simulink model "ClosedLoop_Kernel_RBMCntrl_1A"  (R2023b)
settings: Solver=ode4  StartTime=0.0  StopTime=TMax  FixedStep=DT  MaxStep=DT  RelTol=1e-3  EnableMultiTasking=on
values from neighbouring files (symbols this model uses):
  AirfoilCommand = zeros(1,3)'    [openFASTinit.m]    (also in openFASTinit_v2.m)
  Azimuth_index = 1    [openFASTinit.m]    (also in openFASTinit_v2.m)
  B1N1Alpha_index = 1    [openFASTinit.m]    (also in openFASTinit_v2.m)
  B1N1Cl_index = 1    [openFASTinit.m]    (also in openFASTinit_v2.m)
  B1N1Fl_index = 1    [openFASTinit.m]    (also in openFASTinit_v2.m)
  B1N2Fl_index = 1    [openFASTinit.m]    (also in openFASTinit_v2.m)
  B1N3Fl_index = 1    [openFASTinit.m]    (also in openFASTinit_v2.m)
  B2N1Cl_index = 1    [openFASTinit.m]    (also in openFASTinit_v2.m)
  B2N1Fl_index = 1    [openFASTinit.m]    (also in openFASTinit_v2.m)
  B2N2Fl_index = 1    [openFASTinit.m]    (also in openFASTinit_v2.m)
  B2N3Fl_index = 1    [openFASTinit.m]    (also in openFASTinit_v2.m)
  B3N1Cl_index = 1    [openFASTinit.m]    (also in openFASTinit_v2.m)
  B3N1Fl_index = 1    [openFASTinit.m]    (also in openFASTinit_v2.m)
  B3N2Fl_index = 1    [openFASTinit.m]    (also in openFASTinit_v2.m)
  B3N3Fl_index = 1    [openFASTinit.m]    (also in openFASTinit_v2.m)
  BldPitch1_index = 1    [openFASTinit.m]    (also in openFASTinit_v2.m)
  BldPitch2_index = 1    [openFASTinit.m]    (also in openFASTinit_v2.m)
  BldPitch3_index = 1    [openFASTinit.m]    (also in openFASTinit_v2.m)
  CableDelta_Commande = zeros(1,20)'    [openFASTinit.m]    (also in openFASTinit_v2.m)
  CableDelta_dot_Commande = zeros(1,20)'    [openFASTinit.m]    (also in openFASTinit_v2.m)
  DT = str2double((cell_.Cell_line_1))    [Parameters_checking.m]
  ElectTorque = 1000    [openFASTinit.m]    (also in openFASTinit_v2.m = 500)
  GenPwr_index = 1    [openFASTinit.m]    (also in openFASTinit_v2.m)
  GenTorque = 1000    [openFASTinit.m]    (also in openFASTinit_v2.m = 800)
  GenTq_index = 1    [openFASTinit.m]    (also in openFASTinit_v2.m)
  h_sam = block.InputPort(7).Data    [PMC_kernel.m]
  PtfmPitch_index = 1    [openFASTinit.m]    (also in openFASTinit_v2.m)
  PtfmRoll_index = 1    [openFASTinit.m]    (also in openFASTinit_v2.m)
  PtfmYaw_index = 1    [openFASTinit.m]    (also in openFASTinit_v2.m)
  RootMyb1_index = 1    [openFASTinit.m]    (also in openFASTinit_v2.m)
  RootMyb2_index = 1    [openFASTinit.m]    (also in openFASTinit_v2.m)
  RootMyb3_index = 1    [openFASTinit.m]    (also in openFASTinit_v2.m)
  RootMyc1_index = 1    [openFASTinit.m]    (also in openFASTinit_v2.m)
  RootMyc2_index = 1    [openFASTinit.m]    (also in openFASTinit_v2.m)
  RootMyc3_index = 1    [openFASTinit.m]    (also in openFASTinit_v2.m)
  RotSpeed_index = 1    [openFASTinit.m]    (also in openFASTinit_v2.m)
  ShaftBreaking = 0    [openFASTinit.m]    (also in openFASTinit_v2.m)
  Wind1VelX_index = 1    [openFASTinit.m]    (also in openFASTinit_v2.m)
  YawPosition = 0    [openFASTinit.m]    (also in openFASTinit_v2.m)
  YawRate = 0    [openFASTinit.m]    (also in openFASTinit_v2.m)
undefined symbols (not defined in the file or in its folder): Filter_K, IO_gain, K_alpha_1, K_beta_1, K_divide_1, Kint_1, Kp_1, ratePitchLimit
libraries: cstblocks x4, dspsrcs4 x1
settings Model: Creator=bjonkman  LastModifiedBy=lincoln
settings SolverCC: AlgebraicLoopSolver=TrustRegion
settings DataIOCC: SaveFormat=Array  SignalLoggingSaveFormat=ModelDataLogs  SaveOutput=off  SaveTime=off  ReturnWorkspaceOutputs=off  SignalLoggingName=sigsOut
settings OptimizationCC: ReuseModelBlockBuffer=off  ExpressionDepthLimit=2147483647  LifeSpan=inf
settings DebuggingCC: SaveWithParameterizedLinksMsg=none  UnderspecifiedInitializationDetection=Classic  MergeDetectMultiDrivingBlocksExec=none  SignalResolutionControl=TryResolveAllWithWarning  MultiTaskDSMMsg=warning  MultiTaskCondExecSysMsg=none  FcnCallInpInsideContextMsg=warning  UnconnectedInputMsg=warning  UnconnectedOutputMsg=warning  UnconnectedLineMsg=warning  StateNameClashWarn=warning  SFUnexpectedBacktrackingDiag=warning  SFNoUnconditionalDefaultTransitionDiag=warning  SFExecutionAtInitializationDiag=none  ArithmeticOperatorsInVariantConditions=warning
settings HardwareCC: ProdBitPerPointer=32  ProdBitPerSizeT=32  ProdBitPerPtrDiffT=32  ProdLargestAtomicFloat=None  ProdIntDivRoundTo=Undefined  ProdEndianess=Unspecified  ProdWordSize=32  ProdHWDeviceType=32-bit Generic  TargetUnknown=on
settings ModelReferenceCC: EnableRefExpFcnMdlSchedulingChecks=on  PropagateSignalLabelsOutOfModel=off
settings SFSimCC: SimUseLocalCustomCode=off  CustomCodeUndefinedFunction=UseInterfaceOnly
settings RTWCC: RTWUseLocalCustomCode=off  DLArmComputeVersion=19.05
settings CodeAppCC: StateflowObjectComments=on
settings GRTTargetCC: TargetLangStandard=C89/C90 (ANSI)  CombineOutputUpdateFcns=off  GRTInterface=on
settings ConfigComp: CovMetricSettings=dw  CovSaveCumulativeToWorkspaceVar=on  CovSaveSingleToWorkspaceVar=on  CovExternalEMLEnable=off

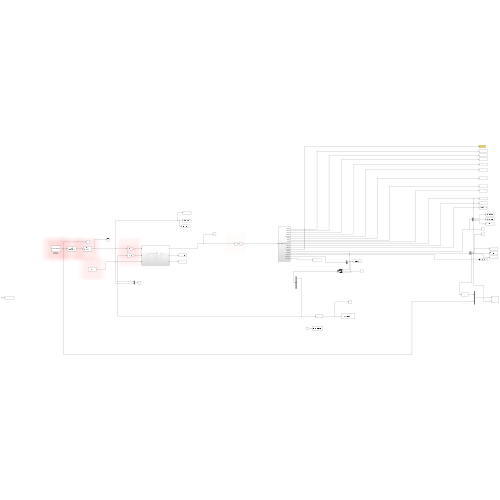
[thumbnail: Simulink's stored preview of the top-level diagram]
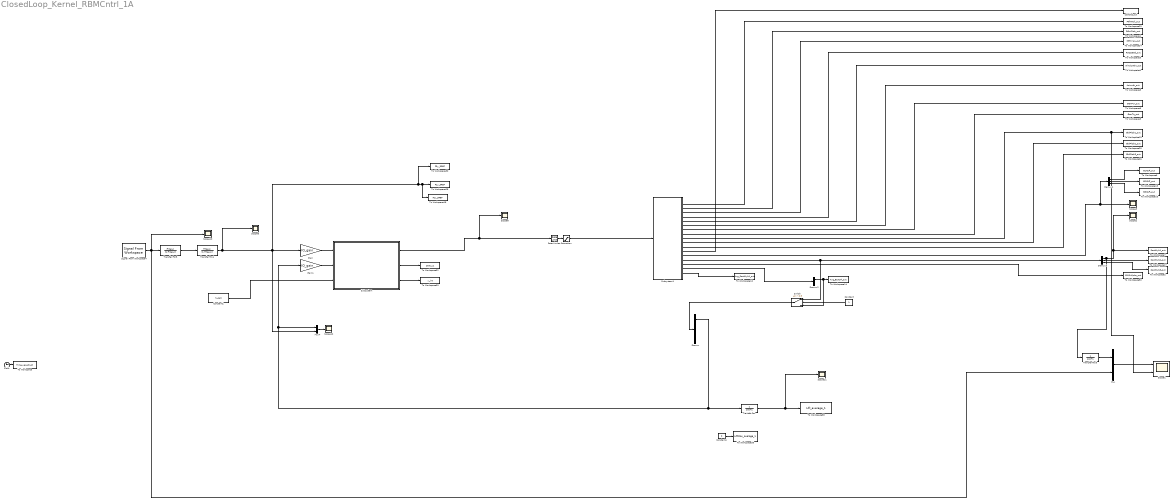
== system ClosedLoop_Kernel_RBMCntrl_1A ==
  Clock : Clock
  Constant : Constant
  Constant1 : Constant  Value=h_sam
  Constant4 : Constant  Value=0
  Demux{,1..3} (4 alike) : Demux  Outputs=3
  Gain : Gain  Gain=IO_gain
  Gain1 : Gain  Gain=IO_gain
  Mux : Mux  Inputs=2
  Mux4 : Mux  Inputs=2
  Rate Limiter : RateLimiter  RisingSlewLimit=ratePitchLimit  FallingSlewLimit=-ratePitchLimit  SampleTimeMode=inherited
  Saturation : Saturate  UpperLimit=0.6  LowerLimit=0
  Scope1 : Scope  NumInputPorts=2
  Scope{2..3,6,8,10..12} (7 alike) : Scope
  Signal From Workspace4 : dspsrcs4/Signal From Workspace  X=TrajectoryReference  Ts=DT  nsamps=1  OutputAfterFinalValue=Setting to zero  ignoreOrWarnInputAndFrameLengths=off  OutputFrames=off
  Subsystem : Subsystem
  Subsystem1 : Subsystem
  Switch : Switch  Criteria=u2 > Threshold  Threshold=0.5  SaturateOnIntegerOverflow=off  InputSameDT=off
  To Workspace : ToWorkspace  VariableName=Time_vec_struct  SaveFormat=Structure With Time  SampleTime=-1
  To Workspace1 : ToWorkspace  VariableName=PtfmPitch_out  SaveFormat=Timeseries  SampleTime=-1
  To Workspace12 : ToWorkspace  VariableName=Avg_RootMyb1_out  SaveFormat=Timeseries  SampleTime=-1
  To Workspace13 : ToWorkspace  VariableName=BldPitch1_out  SaveFormat=Timeseries  SampleTime=-1
  To Workspace14 : ToWorkspace  VariableName=Avg_B1N1Fl_out  SaveFormat=Timeseries  SampleTime=-1
  To Workspace15 : ToWorkspace  VariableName=B2N1Fl_out  SaveFormat=Timeseries  SampleTime=-1
  To Workspace16 : ToWorkspace  VariableName=B3N1Fl_out  SaveFormat=Timeseries  SampleTime=-1
  To Workspace17 : ToWorkspace  VariableName=RootMyb2_out  SaveFormat=Timeseries  SampleTime=-1
  To Workspace18 : ToWorkspace  VariableName=F2y_3REF  SampleTime=-1
  To Workspace2 : ToWorkspace  VariableName=RootMyb3_out  SaveFormat=Timeseries  SampleTime=-1
  To Workspace23 : ToWorkspace  VariableName=PtfmRoll_out  SaveFormat=Timeseries  SampleTime=-1
  To Workspace24 : ToWorkspace  VariableName=PtfmYaw_out  SaveFormat=Timeseries  SampleTime=-1
  To Workspace25 : ToWorkspace  VariableName=BldPitch2_out  SaveFormat=Timeseries  SampleTime=-1
  To Workspace26 : ToWorkspace  VariableName=BldPitch3_out  SaveFormat=Timeseries  SampleTime=-1
  To Workspace28 : ToWorkspace  VariableName=F1y_3REF  SampleTime=-1
  To Workspace3 : ToWorkspace  VariableName=RotSpeed_out  SaveFormat=Timeseries  SampleTime=-1
  To Workspace30 : ToWorkspace  VariableName=F3y_3REF  SampleTime=-1
  To Workspace32 : ToWorkspace  VariableName=para_u1  SampleTime=-1
  To Workspace33 : ToWorkspace  VariableName=y_int  SampleTime=-1
  To Workspace35 : ToWorkspace  VariableName=LiftMax_average_1  SaveFormat=Timeseries  SampleTime=-1
  To Workspace38 : ToWorkspace  VariableName=Lift_average_1  SaveFormat=Timeseries  SampleTime=-1
  To Workspace4 : ToWorkspace  VariableName=Wind1VelX_out  SaveFormat=Timeseries  SampleTime=-1
  To Workspace5 : ToWorkspace  VariableName=Azimuth_out  SaveFormat=Timeseries  SampleTime=-1
  To Workspace50 : ToWorkspace  VariableName=B1N1Alpha_out  SaveFormat=Timeseries  SampleTime=-1
  To Workspace6 : ToWorkspace  VariableName=B1N1Fl_out  SaveFormat=Timeseries  SampleTime=-1
  To Workspace7 : ToWorkspace  VariableName=RootMyb1_out  SaveFormat=Timeseries  SampleTime=-1
  To Workspace8 : ToWorkspace  VariableName=GenPwr_out  SaveFormat=Timeseries  SampleTime=-1
  To Workspace9 : ToWorkspace  VariableName=GenTq_out  SaveFormat=Timeseries  SampleTime=-1
  Transfer Fcn : TransferFcn  Denominator=[10 1]
  Transfer Fcn3 : TransferFcn  Denominator=[10 1]
  Transfer Fcn4 : TransferFcn  Numerator=Filter_K  Denominator=[1 Filter_K]
  Transfer Fcn5 : TransferFcn  Numerator=Filter_K  Denominator=[1 Filter_K]
  qdotdot_out : ToWorkspace  VariableName=OutputChannels  SampleTime=-1
  wires:
  Clock/1 -> To Workspace/1
  Constant1/1 -> Subsystem/3(In3)
  Gain/1 -> Subsystem/1(In1)
  Gain1/1 -> Subsystem/2(In2)
  Subsystem/2(Out2) -> To Workspace32/1
  Subsystem/3(Out3) -> To Workspace33/1
  Mux4/1 -> Scope12/1
  Constant4/1 -> To Workspace35/1
  Demux/1 -> Gain1/1, Mux4/1, Transfer Fcn/1
  Transfer Fcn5/1 -> Transfer Fcn4/1
  Rate Limiter/1 -> Saturation/1
  Transfer Fcn/1 -> Scope11/1, To Workspace38/1
  Transfer Fcn4/1 -> Scope6/1, Mux4/2, Gain/1, To Workspace30/1, To Workspace18/1, To Workspace28/1
  Subsystem1/5(Wind1VelX) -> To Workspace4/1
  Subsystem1/12(Out_States) -> qdotdot_out/1
  Subsystem1/2(PtfmPitch) -> To Workspace1/1
  Subsystem1/1(PtfmRoll) -> To Workspace23/1
  Subsystem1/6(Azimuth) -> To Workspace5/1
  Demux3/1 -> Transfer Fcn3/1, Scope2/1, To Workspace7/1
  Subsystem1/14(RootMyb) -> Switch/1, Demux3/1
  Subsystem1/15(B1N1Alpha) -> To Workspace50/1
  Subsystem1/8(GenTq) -> To Workspace9/1
  Subsystem1/10(BldPitch2) -> To Workspace25/1
  Saturation/1 -> Subsystem1/1(TrajectoryReference)
  Subsystem1/4(RotSpeed) -> To Workspace3/1
  Subsystem1/9(BldPitch1) -> To Workspace13/1, Scope1/2
  Demux1/1 -> To Workspace6/1
  Subsystem1/16(Avg_BxN1Fl) -> Demux2/1
  Subsystem1/7(GenPwr) -> To Workspace8/1
  Subsystem1/3(PtfmYaw) -> To Workspace24/1
  Subsystem1/17(Avg_MYb1) -> To Workspace12/1
  Subsystem1/13(BxN1Fl) -> Demux1/1, Scope3/1
  Demux1/2 -> To Workspace15/1
  Demux1/3 -> To Workspace16/1
  Demux3/2 -> To Workspace17/1
  Demux3/3 -> To Workspace2/1
  Subsystem1/11(BldPitch3) -> To Workspace26/1
  Signal From Workspace4/1 -> Mux/2, Scope10/1, Transfer Fcn5/1
  Subsystem/1(Out1) -> Rate Limiter/1, Scope8/1
  Mux/1 -> Scope1/1
  Transfer Fcn3/1 -> Mux/1
  Demux2/1 -> Switch/3, To Workspace14/1
  Constant/1 -> Switch/2
  Switch/1 -> Demux/1

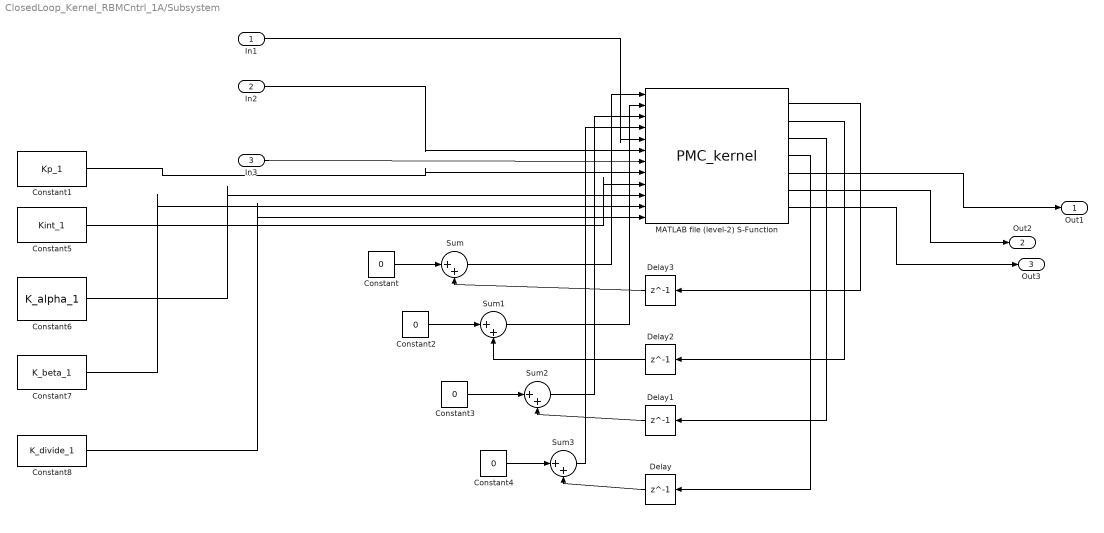
== system ClosedLoop_Kernel_RBMCntrl_1A/Subsystem ==
  In1 : Inport
  In2 : Inport  Port=2
  In3 : Inport  Port=3
  Constant{,2..4} (4 alike) : Constant  Value=0
  Constant1 : Constant  Value=Kp_1
  Constant5 : Constant  Value=Kint_1
  Constant6 : Constant  Value=K_alpha_1
  Constant7 : Constant  Value=K_beta_1
  Constant8 : Constant  Value=K_divide_1
  Delay{,1..3} (4 alike) : Delay  DelayLength=1  InitialCondition=0
  MATLAB file (level-2) S-Function : M-S-Function  FunctionName=PMC_kernel  mask(S-function: msfcn_times_two){}
      mask help: This is a level-2 MATLAB file S-function which multiply input by two.
      mask Display:
      | plot([0 1 2 3 4 5 6 5 4 3 2 1 0 0],[0 .5 1 1.5 2 2.5 3 3.5 4 4.5 5 5.5 6 0]);
      | disp('2      ');
  Sum{,1..3} (4 alike) : Sum  Inputs=|++
  Out1 : Outport
  Out2 : Outport  Port=2
  Out3 : Outport  Port=3
  wires:
  Constant4/1 -> Sum3/1
  In3/1 -> MATLAB file (level-2) S-Function/7
  Sum1/1 -> MATLAB file (level-2) S-Function/2
  Sum/1 -> MATLAB file (level-2) S-Function/1
  MATLAB file (level-2) S-Function/3 -> Delay1/1
  Delay1/1 -> Sum2/2
  MATLAB file (level-2) S-Function/2 -> Delay2/1
  In2/1 -> MATLAB file (level-2) S-Function/6
  In1/1 -> MATLAB file (level-2) S-Function/5
  Sum2/1 -> MATLAB file (level-2) S-Function/3
  Delay/1 -> Sum3/2
  Sum3/1 -> MATLAB file (level-2) S-Function/4
  MATLAB file (level-2) S-Function/4 -> Delay/1
  Constant3/1 -> Sum2/1
  MATLAB file (level-2) S-Function/5 -> Out1/1
  Constant2/1 -> Sum1/1
  Delay3/1 -> Sum/2
  Constant/1 -> Sum/1
  Delay2/1 -> Sum1/2
  MATLAB file (level-2) S-Function/1 -> Delay3/1
  Constant1/1 -> MATLAB file (level-2) S-Function/8
  Constant5/1 -> MATLAB file (level-2) S-Function/9
  Constant6/1 -> MATLAB file (level-2) S-Function/10
  Constant7/1 -> MATLAB file (level-2) S-Function/11
  Constant8/1 -> MATLAB file (level-2) S-Function/12
  MATLAB file (level-2) S-Function/6 -> Out2/1
  MATLAB file (level-2) S-Function/7 -> Out3/1

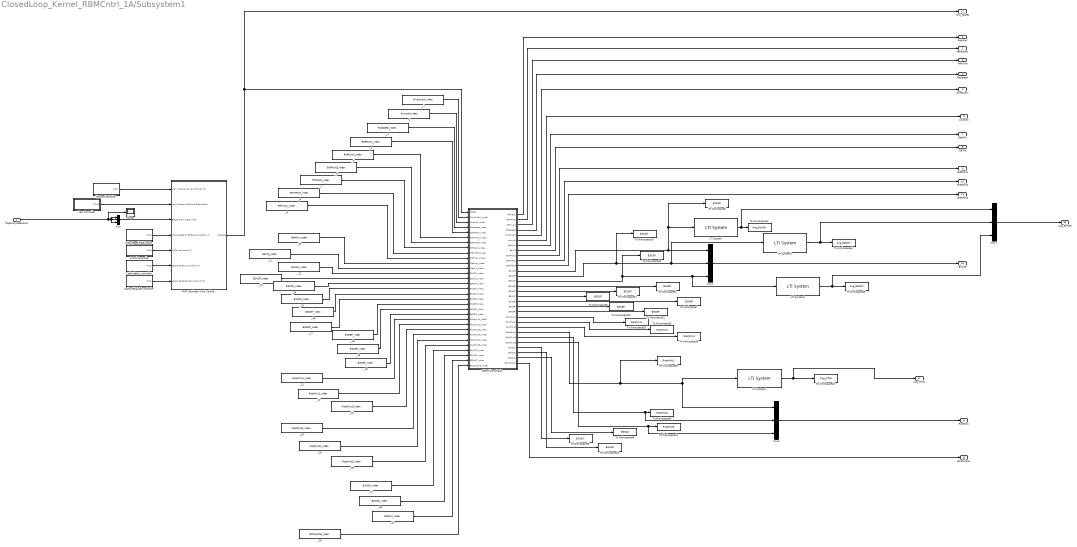
== system ClosedLoop_Kernel_RBMCntrl_1A/Subsystem1 ==
  TrajectoryReference : Inport
  -2 : Constant  Value=Azimuth_index
  AirFoil Controller : Subsystem
  Cable deltaL controller : Subsystem
  Cable deltaLdot controller : Subsystem
  FAST Nonlinear Wind Turbine : Subsystem  mask(FAST Nonlinear Wind Turbine){}
      mask help: This block contains the FAST S-Function.
      mask init:
      | clear FAST_SFunc
  High-Speed Shaft Brake : Subsystem
  LTI System : cstblocks/LTI System  sys=ss(-Filter_K, Filter_K, 1, 0)  IC=IC_lift_output_filter  PadeOrder=0
  LTI System1 : cstblocks/LTI System  sys=ss(-Filter_K, Filter_K, 1, 0)  IC=IC_RBM_output_filter  PadeOrder=0
  LTI System2 : cstblocks/LTI System  sys=ss(-Filter_K, Filter_K, 1, 0)  IC=IC_lift_output_filter  PadeOrder=0
  LTI System3 : cstblocks/LTI System  sys=ss(-Filter_K, Filter_K, 1, 0)  IC=IC_lift_output_filter  PadeOrder=0
  Mux{,1..3} (4 alike) : Mux  Inputs=3
  Scope : Scope
  Select the outputs : MATLAB Function  TreatAsAtomicUnit=on
  To Workspace16 : ToWorkspace  VariableName=B2N1Fl  SaveFormat=Timeseries  SampleTime=-1
  To Workspace17 : ToWorkspace  VariableName=B2N2Fl  SaveFormat=Timeseries  SampleTime=-1
  To Workspace19 : ToWorkspace  VariableName=B3N2Fl  SaveFormat=Timeseries  SampleTime=-1
  To Workspace20 : ToWorkspace  VariableName=B3N1Fl  SaveFormat=Timeseries  SampleTime=-1
  To Workspace21 : ToWorkspace  VariableName=B2N3Fl  SaveFormat=Timeseries  SampleTime=-1
  To Workspace22 : ToWorkspace  VariableName=B3N3Fl  SaveFormat=Timeseries  SampleTime=-1
  To Workspace29 : ToWorkspace  VariableName=RootMyc1  SaveFormat=Timeseries  SampleTime=-1
  To Workspace35 : ToWorkspace  VariableName=RootMyc2  SaveFormat=Timeseries  SampleTime=-1
  To Workspace38 : ToWorkspace  VariableName=RootMyc3  SaveFormat=Timeseries  SampleTime=-1
  To Workspace39 : ToWorkspace  VariableName=RootMyb1  SaveFormat=Timeseries  SampleTime=-1
  To Workspace40 : ToWorkspace  VariableName=RootMyb2  SaveFormat=Timeseries  SampleTime=-1
  To Workspace41 : ToWorkspace  VariableName=RootMyb3  SaveFormat=Timeseries  SampleTime=-1
  To Workspace42 : ToWorkspace  VariableName=Avg_B1N1Fl  SaveFormat=Timeseries  SampleTime=-1
  To Workspace43 : ToWorkspace  VariableName=Avg_MYb1  SaveFormat=Timeseries  SampleTime=-1
  To Workspace44 : ToWorkspace  VariableName=Avg_B2N1Fl  SaveFormat=Timeseries  SampleTime=-1
  To Workspace45 : ToWorkspace  VariableName=Avg_B3N1Fl  SaveFormat=Timeseries  SampleTime=-1
  To Workspace46 : ToWorkspace  VariableName=B1N1Cl  SaveFormat=Timeseries  SampleTime=-1
  To Workspace48 : ToWorkspace  VariableName=B2N1Cl  SaveFormat=Timeseries  SampleTime=-1
  To Workspace49 : ToWorkspace  VariableName=B3N1Cl  SaveFormat=Timeseries  SampleTime=-1
  To Workspace5 : ToWorkspace  VariableName=B1N1Fl  SaveFormat=Timeseries  SampleTime=-1
  To Workspace6 : ToWorkspace  VariableName=B1N2Fl  SaveFormat=Timeseries  SampleTime=-1
  To Workspace7 : ToWorkspace  VariableName=B1N3Fl  SaveFormat=Timeseries  SampleTime=-1
  Torque Controller : Subsystem
  Yaw Controller : Subsystem
  _1 : Constant  Value=Wind1VelX_index
  _10 : Constant  Value=GenPwr_index
  _11 : Constant  Value=GenTq_index
  _12 : Constant  Value=B1N1Fl_index
  _13 : Constant  Value=B2N1Fl_index
  _14 : Constant  Value=B3N1Fl_index
  _15 : Constant  Value=B1N2Fl_index
  _16 : Constant  Value=B2N2Fl_index
  _17 : Constant  Value=B3N2Fl_index
  _18 : Constant  Value=B1N3Fl_index
  _19 : Constant  Value=B2N3Fl_index
  _20 : Constant  Value=B3N3Fl_index
  _21 : Constant  Value=RootMyc1_index
  _22 : Constant  Value=RootMyc2_index
  _23 : Constant  Value=RootMyc3_index
  _24 : Constant  Value=RootMyb1_index
  _25 : Constant  Value=RootMyb2_index
  _26 : Constant  Value=RootMyb3_index
  _27 : Constant  Value=B1N1Cl_index
  _28 : Constant  Value=B2N1Cl_index
  _29 : Constant  Value=B3N1Cl_index
  _3 : Constant  Value=RotSpeed_index
  _30 : Constant  Value=B1N1Alpha_index
  _4 : Constant  Value=BldPitch1_index
  _5 : Constant  Value=BldPitch2_index
  _6 : Constant  Value=BldPitch3_index
  _7 : Constant  Value=PtfmRoll_index
  _8 : Constant  Value=PtfmPitch_index
  _9 : Constant  Value=PtfmYaw_index
  PtfmRoll : Outport
  PtfmPitch : Outport  Port=2
  PtfmYaw : Outport  Port=3
  RotSpeed : Outport  Port=4
  Wind1VelX : Outport  Port=5
  Azimuth : Outport  Port=6
  GenPwr : Outport  Port=7
  GenTq : Outport  Port=8
  BldPitch1 : Outport  Port=9
  BldPitch2 : Outport  Port=10
  BldPitch3 : Outport  Port=11
  Out_States : Outport  Port=12
  BxN1Fl : Outport  Port=13
  RootMyb : Outport  Port=14
  B1N1Alpha : Outport  Port=15
  Avg_BxN1Fl : Outport  Port=16
  Avg_MYb1 : Outport  Port=17
  wires:
  Mux3/1 -> RootMyb/1
  Select the outputs/8(GenTq) -> GenTq/1
  Select the outputs/3(PtfmYaw) -> PtfmYaw/1
  Select the outputs/7(GenPwr) -> GenPwr/1
  Select the outputs/1(PtfmRoll) -> PtfmRoll/1
  Select the outputs/27(B1N1Cl) -> To Workspace46/1
  _3/1 -> Select the outputs/4(RotSpeed_index)
  Select the outputs/15(B1N2Fl) -> To Workspace6/1
  LTI System3/1 -> Mux1/3, To Workspace45/1
  Select the outputs/29(B3N1Cl) -> To Workspace49/1
  _5/1 -> Select the outputs/6(BldPitch2_index)
  _7/1 -> Select the outputs/8(PtfmRoll_index)
  -2/1 -> Select the outputs/3(Azimuth_index)
  _22/1 -> Select the outputs/23(RootMyc2_index)
  _10/1 -> Select the outputs/11(GenPwr_index)
  FAST Nonlinear Wind Turbine/1(OutData) -> Select the outputs/1(states), Out_States/1
  Select the outputs/10(BldPitch2) -> BldPitch2/1
  _19/1 -> Select the outputs/20(B2N3Fl_index)
  Select the outputs/13(B2N1Fl) -> LTI System2/1, Mux2/2, To Workspace16/1
  Select the outputs/6(Azimuth) -> Azimuth/1
  Select the outputs/25(RootMyb2) -> Mux3/2, To Workspace40/1
  Cable deltaLdot controller/1(Out1) -> FAST Nonlinear Wind Turbine/7(Cable deltaLdot command (m/s))
  Select the outputs/30(B1N1Alpha) -> B1N1Alpha/1
  Select the outputs/11(BldPitch3) -> BldPitch3/1
  Select the outputs/20(B3N3Fl) -> To Workspace22/1
  _30/1 -> Select the outputs/31(B1N1Alpha_index)
  High-Speed Shaft Brake/1(Out1) -> FAST Nonlinear Wind Turbine/4(High-Speed Shaft Braking Fraction (-))
  Select the outputs/21(RootMyc1) -> To Workspace29/1
  _13/1 -> Select the outputs/14(B2N1Fl_index)
  _12/1 -> Select the outputs/13(B1N1Fl_index)
  _6/1 -> Select the outputs/7(BldPitch3_index)
  Select the outputs/26(RootMyb3) -> Mux3/3, To Workspace41/1
  LTI System1/1 -> Avg_MYb1/1, To Workspace43/1
  _8/1 -> Select the outputs/9(PtfmPitch_index)
  LTI System/1 -> Mux1/1, To Workspace42/1
  _1/1 -> Select the outputs/2(Wind1VelX_index)
  Torque Controller/1(Out1) -> FAST Nonlinear Wind Turbine/1(Gen. Torque (Nm) and Power (W))
  _9/1 -> Select the outputs/10(PtfmYaw_index)
  _25/1 -> Select the outputs/26(RootMyb2_index)
  Mux2/1 -> BxN1Fl/1
  _29/1 -> Select the outputs/30(B3N1Cl_index)
  Select the outputs/17(B3N2Fl) -> To Workspace19/1
  Select the outputs/19(B2N3Fl) -> To Workspace21/1
  _20/1 -> Select the outputs/21(B3N3Fl_index)
  _4/1 -> Select the outputs/5(BldPitch1_index)
  Select the outputs/14(B3N1Fl) -> To Workspace20/1, LTI System3/1, Mux2/3
  _24/1 -> Select the outputs/25(RootMyb1_index)
  Select the outputs/24(RootMyb1) -> To Workspace39/1, Mux3/1, LTI System1/1
  Select the outputs/16(B2N2Fl) -> To Workspace17/1
  _15/1 -> Select the outputs/16(B1N2Fl_index)
  _18/1 -> Select the outputs/19(B1N3Fl_index)
  Select the outputs/5(Wind1VelX) -> Wind1VelX/1
  _23/1 -> Select the outputs/24(RootMyc3_index)
  _21/1 -> Select the outputs/22(RootMyc1_index)
  Select the outputs/2(PtfmPitch) -> PtfmPitch/1
  TrajectoryReference/1 -> Scope/1, Mux/1, Mux/3, Mux/2
  Yaw Controller/1(Out1) -> FAST Nonlinear Wind Turbine/2(Yaw Position (rad) and Rate (rad/s))
  Mux/1 -> FAST Nonlinear Wind Turbine/3(Blade Pitch Angles (rad))
  Select the outputs/12(B1N1Fl) -> To Workspace5/1, LTI System/1, Mux2/1
  Select the outputs/23(RootMyc3) -> To Workspace38/1
  _17/1 -> Select the outputs/18(B3N2Fl_index)
  Select the outputs/9(BldPitch1) -> BldPitch1/1
  _28/1 -> Select the outputs/29(B2N1Cl_index)
  _11/1 -> Select the outputs/12(GenTq_index)
  Select the outputs/4(RotSpeed) -> RotSpeed/1
  Select the outputs/22(RootMyc2) -> To Workspace35/1
  Cable deltaL controller/1(Out1) -> FAST Nonlinear Wind Turbine/6(Cable deltaL command (m))
  _14/1 -> Select the outputs/15(B3N1Fl_index)
  _27/1 -> Select the outputs/28(B1N1Cl_index)
  AirFoil Controller/1(Out1) -> FAST Nonlinear Wind Turbine/5(AirFoil command (-))
  _26/1 -> Select the outputs/27(RootMyb3_index)
  _16/1 -> Select the outputs/17(B2N2Fl_index)
  Select the outputs/28(B2N1Cl) -> To Workspace48/1
  Select the outputs/18(B1N3Fl) -> To Workspace7/1
  LTI System2/1 -> Mux1/2, To Workspace44/1
  Mux1/1 -> Avg_BxN1Fl/1

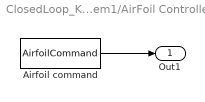
== system ClosedLoop_Kernel_RBMCntrl_1A/Subsystem1/AirFoil Controller ==
  Airfoil command : Constant  Value=AirfoilCommand
  Out1 : Outport
  wires:
  Airfoil command/1 -> Out1/1

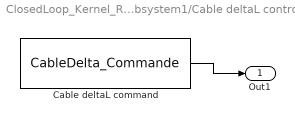
== system ClosedLoop_Kernel_RBMCntrl_1A/Subsystem1/Cable deltaL controller ==
  Cable deltaL command : Constant  Value=CableDelta_Commande
  Out1 : Outport
  wires:
  Cable deltaL command/1 -> Out1/1

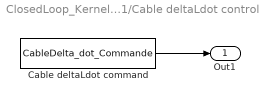
== system ClosedLoop_Kernel_RBMCntrl_1A/Subsystem1/Cable deltaLdot controller ==
  Cable deltaLdot command : Constant  Value=CableDelta_dot_Commande
  Out1 : Outport
  wires:
  Cable deltaLdot command/1 -> Out1/1

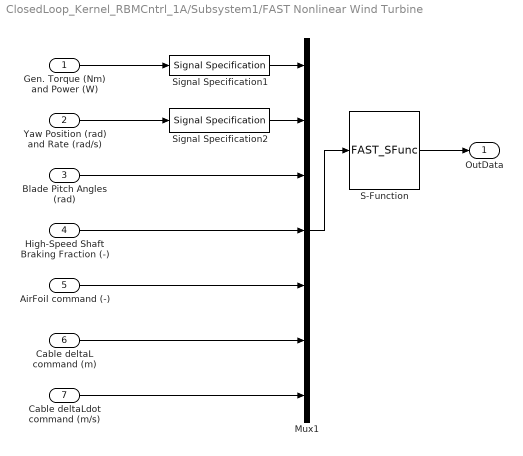
== system ClosedLoop_Kernel_RBMCntrl_1A/Subsystem1/FAST Nonlinear Wind Turbine ==
  Gen. Torque (Nm) and Power (W) : Inport
  Yaw Position (rad) and Rate (rad/s) : Inport  Port=2
  Blade Pitch Angles (rad) : Inport  Port=3
  High-Speed Shaft Braking Fraction (-) : Inport  Port=4
  AirFoil command (-) : Inport  Port=5
  Cable deltaL command (m) : Inport  Port=6
  Cable deltaLdot command (m/s) : Inport  Port=7
  Mux1 : Mux  Inputs=7
  S-Function : S-Function  FunctionName=FAST_SFunc  Parameters=FAST_InputFileName, TMax, 0  SFunctionDeploymentMode=off  EnableBusSupport=off
  Signal Specification1 : SignalSpecification  OutDataTypeStr=double  Dimensions=2
  Signal Specification2 : SignalSpecification  OutDataTypeStr=double  Dimensions=2
  OutData : Outport
  wires:
  Gen. Torque (Nm) and Power (W)/1 -> Signal Specification1/1
  S-Function/1 -> OutData/1
  Mux1/1 -> S-Function/1
  Blade Pitch Angles (rad)/1 -> Mux1/3
  Yaw Position (rad) and Rate (rad/s)/1 -> Signal Specification2/1
  Signal Specification1/1 -> Mux1/1
  Signal Specification2/1 -> Mux1/2
  High-Speed Shaft Braking Fraction (-)/1 -> Mux1/4
  AirFoil command (-)/1 -> Mux1/5
  Cable deltaL command (m)/1 -> Mux1/6
  Cable deltaLdot command (m/s)/1 -> Mux1/7

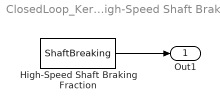
== system ClosedLoop_Kernel_RBMCntrl_1A/Subsystem1/High-Speed Shaft Brake ==
  High-Speed Shaft Braking Fraction : Constant  Value=ShaftBreaking
  Out1 : Outport
  wires:
  High-Speed Shaft Braking Fraction/1 -> Out1/1

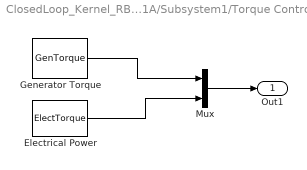
== system ClosedLoop_Kernel_RBMCntrl_1A/Subsystem1/Torque Controller ==
  Electrical Power : Constant  Value=ElectTorque
  Generator Torque : Constant  Value=GenTorque
  Mux : Mux  Inputs=2
  Out1 : Outport
  wires:
  Mux/1 -> Out1/1
  Generator Torque/1 -> Mux/1
  Electrical Power/1 -> Mux/2

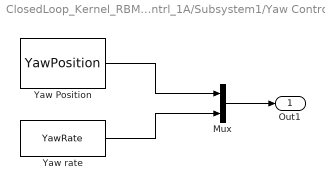
== system ClosedLoop_Kernel_RBMCntrl_1A/Subsystem1/Yaw Controller ==
  Mux : Mux  Inputs=2
  Yaw Position : Constant  Value=YawPosition
  Yaw rate : Constant  Value=YawRate
  Out1 : Outport
  wires:
  Mux/1 -> Out1/1
  Yaw Position/1 -> Mux/1
  Yaw rate/1 -> Mux/2

== matlab function ClosedLoop_Kernel_RBMCntrl_1A/Subsystem1/Select the outputs ==
  data: PtfmRoll output; PtfmPitch output; PtfmYaw output; RotSpeed output; states input; Wind1VelX output; Azimuth output; GenPwr output; GenTq output; BldPitch1 output; BldPitch2 output; BldPitch3 output; Wind1VelX_index input; Azimuth_index input; RotSpeed_index input; BldPitch1_index input; BldPitch2_index input; BldPitch3_index input; PtfmRoll_index input; PtfmPitch_index input; PtfmYaw_index input; GenPwr_index input; GenTq_index input; B1N1Fl_index input; B2N1Fl_index input; B3N1Fl_index input; B1N2Fl_index input; B2N2Fl_index input; B3N2Fl_index input; B1N3Fl_index input; B2N3Fl_index input; B3N3Fl_index input; B1N1Fl output; B2N1Fl output; B3N1Fl output; B1N2Fl output; B2N2Fl output; B3N2Fl output; B1N3Fl output; B2N3Fl output; B3N3Fl output; RootMyc1 output; RootMyc2 output; RootMyc3 output; RootMyc1_index input; RootMyc2_index input; RootMyc3_index input; RootMyb1_index input; RootMyb2_index input; RootMyb3_index input; RootMyb1 output; RootMyb2 output; RootMyb3 output; B1N1Cl_index input; B2N1Cl_index input; B3N1Cl_index input; B1N1Cl output; B2N1Cl output; B3N1Cl output; B1N1Alpha_index input; B1N1Alpha output
function [PtfmRoll, PtfmPitch, PtfmYaw, ...
            RotSpeed, Wind1VelX, ...
         Azimuth, ...
         GenPwr, GenTq, ...
         BldPitch1, BldPitch2, BldPitch3, ...
         B1N1Fl, B2N1Fl, B3N1Fl, ...
         B1N2Fl, B2N2Fl, B3N2Fl, ...
         B1N3Fl, B2N3Fl, B3N3Fl, ...
         RootMyc1, RootMyc2, RootMyc3, ...
         RootMyb1, RootMyb2, RootMyb3, ...
         B1N1Cl, B2N1Cl, B3N1Cl, B1N1Alpha] = fcn(states, Wind1VelX_index, Azimuth_index, RotSpeed_index, BldPitch1_index, ...
         BldPitch2_index, BldPitch3_index, PtfmRoll_index, PtfmPitch_index, PtfmYaw_index, ...
         GenPwr_index, GenTq_index, ...
         B1N1Fl_index, B2N1Fl_index, B3N1Fl_index, ...
         B1N2Fl_index, B2N2Fl_index, B3N2Fl_index, ...
         B1N3Fl_index, B2N3Fl_index, B3N3Fl_index, ...
         RootMyc1_index, RootMyc2_index, RootMyc3_index, ...
         RootMyb1_index, RootMyb2_index, RootMyb3_index, ...
         B1N1Cl_index, B2N1Cl_index, B3N1Cl_index, B1N1Alpha_index)

% ================== List of outputs

%    Wind1VelX             (m/s)                 InflowWind
%    Wind1VelY             (m/s)                 InflowWind
%    Wind1VelZ             (m/s)                 InflowWind
Wind1VelX = states(Wind1VelX_index); 

%    Azimuth               (deg)                 ElastoDyn 
Azimuth = states(Azimuth_index); 

%    RotSpeed              (rpm)                 ElastoDyn
RotSpeed = states(RotSpeed_index)/(30/pi); 

%    BldPitch1             (deg)                 ElastoDyn
BldPitch1 = states(BldPitch1_index); 
%    BldPitch2             (deg)                 ElastoDyn
BldPitch2 = states(BldPitch2_index); 
%    BldPitch3             (deg)
BldPitch3 = states(BldPitch3_index);

%   PtfmRoll             (deg)                 ElastoDyn
PtfmRoll = states(PtfmRoll_index)/(180/pi); 
%   PtfmPitch            (deg)                 ElastoDyn 
PtfmPitch = states(PtfmPitch_index)/(180/pi); 
%   PtfmYaw             (deg)                 ElastoDyn 
PtfmYaw = states(PtfmYaw_index)/(180/pi);  

%  RootMyb-c1_index
RootMyb1 = states(RootMyb1_index);
RootMyc1 = states(RootMyc1_index);

%  RootMyb-c2_index
RootMyb2 = states(RootMyb2_index);
RootMyc2 = states(RootMyc2_index);

%  RootMyb-c3_index
RootMyb3 = states(RootMyb3_index);
RootMyc3 = states(RootMyc3_index);


%   GenPwr                (kW)                  ServoDyn 
%   GenTq                 (kN-m)                ServoDyn 
GenPwr = states(GenPwr_index);  
GenTq = states(GenTq_index);   


%   B1N1Fl                (N/m)                 AeroDyn 
%   B1N2Fl                (N/m)                 AeroDyn
%   B1N3Fl                (N/m)                 AeroDyn
B1N1Fl = states(B1N1Fl_index); 
B2N1Fl = states(B2N1Fl_index); 
B3N1Fl = states(B3N1Fl_index); 

%   B2N1Fl                (N/m)                 AeroDyn
%   B2N2Fl                (N/m)                 AeroDyn
%   B2N3Fl                (N/m)                 AeroDyn

B1N2Fl = states(B1N2Fl_index); 
B2N2Fl = states(B2N2Fl_index); 
B3N2Fl = states(B3N2Fl_index); 

%   B3N1Fl                (N/m)                 AeroDyn
%   B3N2Fl                (N/m)                 AeroDyn
%   B3N3Fl                (N/m)                 AeroDyn

B1N3Fl = states(B1N3Fl_index); 
B2N3Fl = states(B2N3Fl_index); 
B3N3Fl = states(B3N3Fl_index); 


B1N1Cl = states(B1N1Cl_index);
B2N1Cl = states(B2N1Cl_index);
B3N1Cl = states(B3N1Cl_index);


B1N1Alpha = states(B1N1Alpha_index);
